simulink model "ex1"  (R2015a)
settings: Solver=ode45  StartTime=0.0  StopTime=10.0  RelTol=1e-3
values from neighbouring files (symbols this model uses):
  A = [0 1; -5 -2]    [ex1.m]
  B = [0;1]    [ex1.m]
  C = [1 0]    [ex1.m]
  K = place(A,B,P)    [ex1.m]
settings Model: Creator=Xrisostomos  LastModifiedBy=Xrisostomos

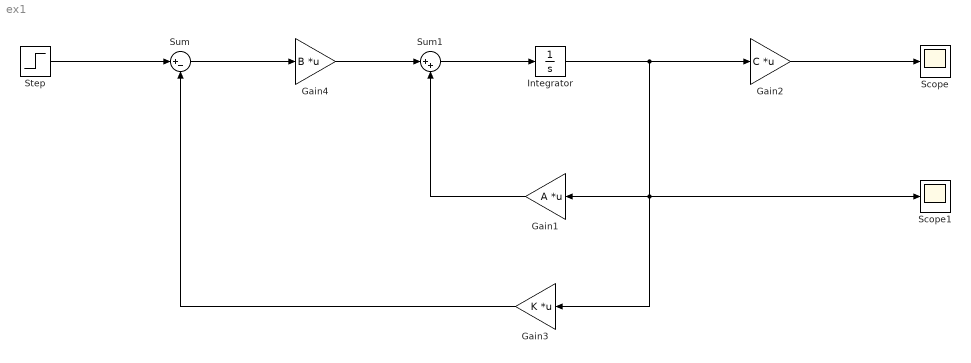
== system ex1 ==
  Gain1 : Gain  Gain=A  Multiplication=Matrix(K*u)
  Gain2 : Gain  Gain=C  Multiplication=Matrix(K*u)
  Gain3 : Gain  Gain=K  Multiplication=Matrix(K*u)
  Gain4 : Gain  Gain=B  Multiplication=Matrix(K*u)
  Integrator : Integrator
  Scope : Scope
  Scope1 : Scope
      settings: TimeRange=10
  Step : Step  SampleTime=0
  Sum : Sum  Inputs=|+-
  Sum1 : Sum  Inputs=|++
  wires:
  Step/1 -> Sum/1
  Sum1/1 -> Integrator/1
  Integrator/1 -> Gain3/1, Gain1/1, Scope1/1, Gain2/1
  Gain3/1 -> Sum/2
  Gain1/1 -> Sum1/2
  Gain2/1 -> Scope/1
  Sum/1 -> Gain4/1
  Gain4/1 -> Sum1/1
